simulink model "PowerOutlet"  (R2020b)
settings: Solver=VariableStepAuto  StartTime=0.0  StopTime=10  RelTol=1e-3
undefined symbols (not defined in the file): sigbuilder_block
settings Model: Creator=99003778  LastModifiedBy=99003778

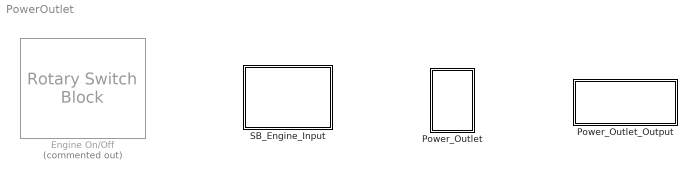
== system PowerOutlet ==
  Engine On/Off : RotarySwitchBlock  Commented=on
      settings: Values={{'Off', 'On'}, [0 1]}
  Power_Outlet : Subsystem
  Power_Outlet_Output : Subsystem
  SB_Engine_Input : Subsystem

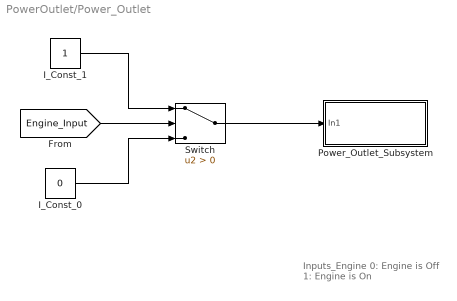
== system PowerOutlet/Power_Outlet ==
  note: Inputs_Engine
      |
      | 0: Engine is Off
      | 1: Engine is On
  I_Const_0 : Constant  Value=0
  I_Const_1 : Constant
  Power_Outlet_Subsystem : Subsystem
  Switch : Switch  Criteria=u2 > Threshold
  wires:
  I_Const_0/1 -> Switch/3
  [Engine_Input] -> Switch/2
  Switch/1 -> Power_Outlet_Subsystem/1(In1)
  I_Const_1/1 -> Switch/1

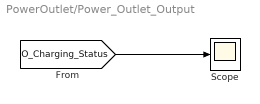
== system PowerOutlet/Power_Outlet_Output ==
  Scope : Scope
  wires:
  [O_Charging_Status] -> Scope/1

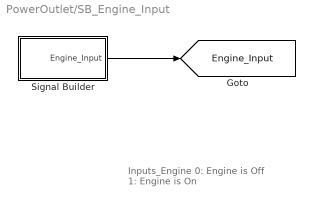
== system PowerOutlet/SB_Engine_Input ==
  note: Inputs_Engine
      |
      | 0: Engine is Off
      | 1: Engine is On
  Signal Builder : Subsystem  Tag=STV Subsys  LoadFcn=sigbuilder_block('load',[197.25 223.5 550.5 359.25 ]);  StartFcn=sigbuilder_block('start');  StopFcn=sigbuilder_block('stop');  ClipboardFcn=sigbuilder_block('clipboard');  mask(Sigbuilder block){tuvar=[0:10]}
      mask help: Simulink:masks:SigbuilderBlock_MD
      mask init:
      | if ~strcmp(get_param(bdroot(gcbh),'SimulationStatus'),'stopped') tuvar = sigbuilder_block('maskInit'); end
      settings: CopyFcn=sigbuilder_block('copy');  DeleteFcn=sigbuilder_block('delete');  ModelCloseFcn=sigbuilder_block('modelClose');  PreSaveFcn=sigbuilder_block('preSave');  PauseFcn=sigbuilder_block('pause');  ContinueFcn=sigbuilder_block('continue');  NameChangeFcn=sigbuilder_block('namechange');  OpenFcn=sigbuilder_block('open',[403.5 199.2 550.5 359.55 ]);  CloseFcn=sigbuilder_block('close');
      mask Display: plot(0, 0, 100, 100,[2, 2, 32, 32, 2], [68, 8, 8, 68, 68],[32, 2], [38, 38], [32, 19, 2],[53, 60, 44], [32, 17, 17, 2],[16, 16, 31, 31]);txt = getActiveGroup(gcbh);text(2, 100, txt,'verticalAlignment', 'top');
  tag scope: Engine_Input=global
  wires:
  Signal Builder/1(Engine_Input) -> [Engine_Input]

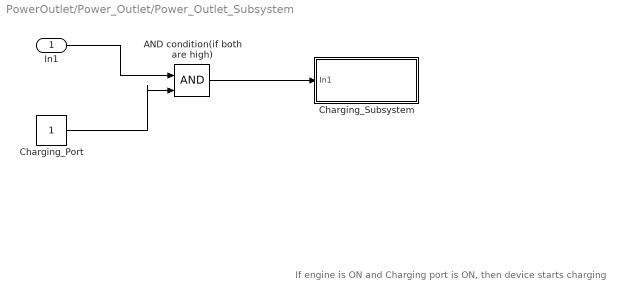
== system PowerOutlet/Power_Outlet/Power_Outlet_Subsystem ==
  note: If engine is ON and Charging port is ON, then device starts charging
  In1 : Inport
  AND condition(if both are high) : Logic  IconShape=distinctive  AllPortsSameDT=off  OutDataTypeStr=boolean
  Charging_Port : Constant
  Charging_Subsystem : Subsystem
  wires:
  In1/1 -> AND condition(if both are high)/1
  Charging_Port/1 -> AND condition(if both are high)/2
  AND condition(if both are high)/1 -> Charging_Subsystem/1(In1)

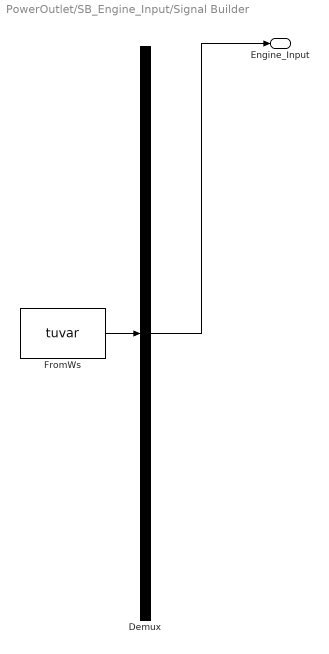
== system PowerOutlet/SB_Engine_Input/Signal Builder ==
  Demux : Demux  Tag=STV Demux  Outputs=1
      settings: DisplayOption=none
  FromWs : FromWorkspace  Tag=STV FromWs  VariableName=tuvar
      SigBuilderData=|
      | common.afterFinalStr = 'Extrapolate'
      | common.sampleTime = 0
      | dataSet.timeRange = [0 10]
      | dataSet.name = 'Group 1'
      | sbobj.Groups.Name = 'Group 1'
      | sbobj.Groups.Signals.Name = 'Engine_Input'
      | sbobj.Groups.Signals.XData = [0 1 2 3 4 5 6 7 8 9 10 11 12 13 14 15 16 17 18 19 20 21 22 23 24 25]
      | sbobj.Groups.Signals.YData = [0 1 1 0 1 1 0 0 0 1 1 1 0 0 1 0 0 1 0 1 0 0 0 1 1 0]
  Engine_Input : Outport  Tag=STV Outport
  wires:
  FromWs/1 -> Demux/1
  Demux/1 -> Engine_Input/1

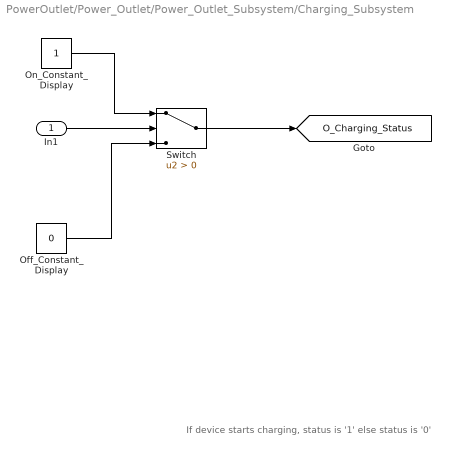
== system PowerOutlet/Power_Outlet/Power_Outlet_Subsystem/Charging_Subsystem ==
  note: If device starts charging, status is '1'
      | else status is '0'
  In1 : Inport
  Off_Constant_Display : Constant  Value=0
  On_Constant_Display : Constant
  Switch : Switch  Criteria=u2 > Threshold
  tag scope: O_Charging_Status=global
  wires:
  In1/1 -> Switch/2
  On_Constant_Display/1 -> Switch/1
  Off_Constant_Display/1 -> Switch/3
  Switch/1 -> [O_Charging_Status]
